simulink model "Test_measurement_script"  (R2019b)
settings: Solver=FixedStepAuto  StartTime=0.0  StopTime=10.0  RelTol=1e-3
PostLoadFcn:
  | if any(exist('dsrtsu_mdlpostloadfcn', 'file') ~= 0), dsrtsu_mdlpostloadfcn('Execute', bdroot); end
values from neighbouring files (symbols this model uses):
  UseUserDefinedBallReference = 1    [LQG_ball.m]    (also in LQG_plate_ball.m; LQR_ball.m; PerformExperiment_CompareModelWithMeasurement.m = 0; Template_PerformExperiment.m = 0)
  UseUserDefinedPlateReference = 1    [LQG_ball.m]    (also in LQG_plate_ball.m; LQR_ball.m; PerformExperiment_CompareModelWithMeasurement.m; Template_PerformExperiment.m = 0)
settings Model: DSRTSU_INTERNAL_RTI_VER=570  DSRTSU_INTERNAL_RTI_TYPE=rti1202  Creator=Duin home  LastModifiedBy=20201073
settings HardwareCC: ProdBitPerPointer=32  ProdBitPerSizeT=32  ProdBitPerPtrDiffT=32  ProdLargestAtomicInteger=Integer  ProdEndianess=BigEndian  ProdWordSize=32  ProdLongLongMode=on  ProdHWDeviceType=Custom Processor->Custom  TargetIntDivRoundTo=Zero  TargetEndianess=BigEndian  TargetHWDeviceType=Custom Processor->Custom
settings SFSimCC: MATLABDynamicMemAlloc=off
settings RTWCC: Description=dSPACE DS1202 Hardware Platform  SystemTargetFile=rti1202.tlc  MakeCommand=make_rti  TemplateMakefile=rti1202.tmf
settings STFCustomTargetCC: ParMdlRefBuildCompliant=on  SystemTargetFile=rti1202.tlc
settings GRTTargetCC: TargetLangStandard=C89/C90 (ANSI)  CompOptLevelCompliant=off  ConcurrentExecutionCompliant=off  CombineOutputUpdateFcns=off  MatFileLogging=off  CPPClassGenCompliant=off  UseToolchainInfoCompliant=off

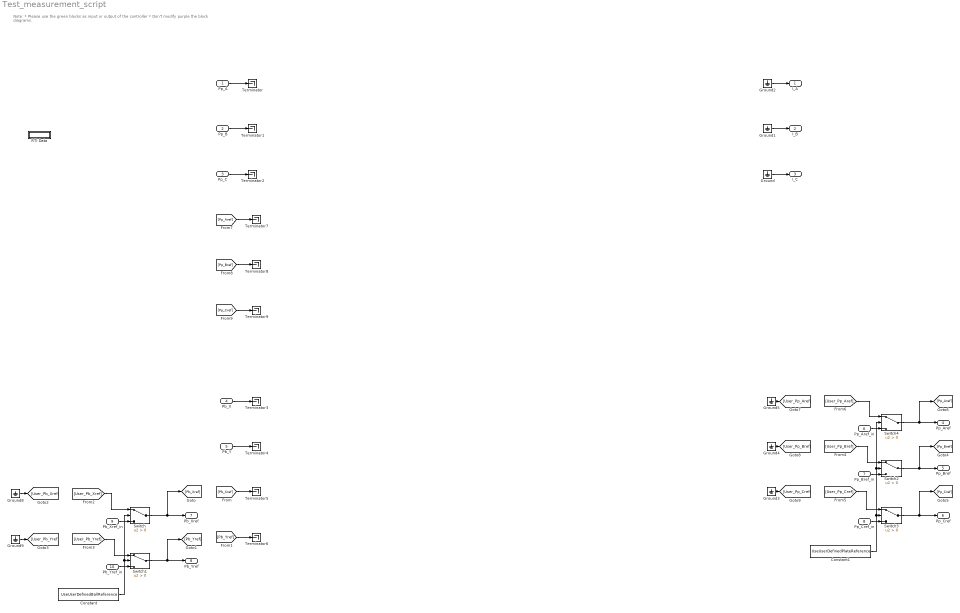
== system Test_measurement_script ==
  note: Note:
      | * Please use the green blocks as input or output of the controller
      | * Don't modify purple the block diagrams.
  Pp_A : Inport
  Pp_B : Inport  Port=2
  Pp_C : Inport  Port=3
  Pb_X : Inport  Port=4
  Pb_Y : Inport  Port=5
  Pp_Aref_in : Inport  Port=6
  Pp_Bref_in : Inport  Port=7
  Pp_Cref_in : Inport  Port=8
  Pb_Xref_in : Inport  Port=9
  Pb_Yref_in : Inport  Port=10
  Constant : Constant  Value=UseUserDefinedBallReference
  Constant1 : Constant  Value=UseUserDefinedPlateReference
  Ground{,1..5,8..9} (8 alike) : Ground
  RTI Data : Subsystem  Tag=struct('RTIDataServer',struct('RTIDataServerVs','2','RTIModelDescription','struct(''main'',''Test_measurement_script'',''sub'',''Test_measurement_script'',''isMp'',0)'))  LoadFcn="if exist('rtidc'), try,  rtidc('DataHostBlockClbLoad', gcbh); catch, disp(['Warning: ''LoadFcn'' for RTI Data block failed: ' lasterr]); end, end,"  mask(RTI_DATA_HOST){}
      mask help:
      | RTI Data Block.
      | This block is used by RTI to store internal model-dependent data.
      | Please keep this block on the root level of the model. Deleting this block will result in data loss.
      |
      | NEVER DELETE OR COPY THIS BLOCK!
      settings: CopyFcn="if exist('rtidc'), try,  rtidc('DataHostBlockClbCopy', gcbh); catch, disp(['Warning: ''CopyFcn'' for RTI Data block failed: ' lasterr]); end, end,"  DeleteFcn="if exist('rtidc'), try,  rtidc('DataHostBlockClbDelete', gcbh); catch, disp(['Warning: ''DeleteFcn'' for RTI Data block failed: ' lasterr]); end, end,"  ModelCloseFcn="if exist('rtidc'), try,  rtidc('DataHostBlockClbModelClose', gcbh); catch, disp(['Warning: ''ModelCloseFcn'' for RTI Data block failed: ' lasterr]); end, end,"  PreSaveFcn="if exist('rtidc'), try,  rtidc('DataHostBlockClbPreSave', gcbh); catch, disp(['Warning: ''PreSaveFcn'' for RTI Data block failed: ' lasterr]); end, end,"  PostSaveFcn="if exist('rtidc'), try,  rtidc('DataHostBlockClbPostSave', gcbh); catch, disp(['Warning: ''PostSaveFcn'' for RTI Data block failed: ' lasterr]); end, end,"  NameChangeFcn="if exist('rtidc'), try,  rtidc('DataHostBlockClbNameChange', gcbh); catch, disp(['Warning: ''NameChangeFcn'' for RTI Data block failed: ' lasterr]); end, end,"
      mask Help:
      | RTI Data Block.
      | This block is used by RTI to store internal model-dependent data.
      | Please keep this block on the root level of the model. Deleting this block will result in data loss.
      | 
      | NEVER DELETE OR COPY THIS BLOCK!
      mask Display:
      | text(0.5, 0.5, 'RTI Data', 'HorizontalAlignment', 'center');
      | plot([1 0]);
  Switch{,1..4} (5 alike) : Switch  Criteria=u2 > Threshold
  Terminator{,1..9} (10 alike) : Terminator
  I_A : Outport
  I_B : Outport  Port=2
  I_C : Outport  Port=3
  Pp_Aref : Outport  Port=4
  Pp_Bref : Outport  Port=5
  Pp_Cref : Outport  Port=6
  Pb_Xref : Outport  Port=7
  Pb_Yref : Outport  Port=8
  wires:
  Pp_A/1 -> Terminator/1
  Pp_B/1 -> Terminator1/1
  Pp_C/1 -> Terminator2/1
  Pb_X/1 -> Terminator3/1
  Pb_Y/1 -> Terminator4/1
  Ground/1 -> I_C/1
  Ground1/1 -> I_B/1
  Ground2/1 -> I_A/1
  Ground3/1 -> [User_Pp_Cref]
  Ground4/1 -> [User_Pp_Bref]
  Ground5/1 -> [User_Pp_Aref]
  Pb_Xref_in/1 -> Switch/3
  Pb_Yref_in/1 -> Switch1/3
  Switch1/1 -> [Pb_Yref], Pb_Yref/1
  Switch/1 -> [Pb_Xref], Pb_Xref/1
  [User_Pb_Xref] -> Switch/1
  [User_Pb_Yref] -> Switch1/1
  Constant/1 -> Switch/2, Switch1/2
  Ground8/1 -> [User_Pb_Xref]
  Ground9/1 -> [User_Pb_Yref]
  [Pb_Yref] -> Terminator6/1
  [Pb_Xref] -> Terminator5/1
  Pp_Bref_in/1 -> Switch2/3
  [User_Pp_Bref] -> Switch2/1
  Switch3/1 -> [Pp_Cref], Pp_Cref/1
  Switch2/1 -> [Pp_Bref], Pp_Bref/1
  Pp_Cref_in/1 -> Switch3/3
  Constant1/1 -> Switch4/2, Switch2/2, Switch3/2
  [User_Pp_Cref] -> Switch3/1
  [User_Pp_Aref] -> Switch4/1
  Pp_Aref_in/1 -> Switch4/3
  Switch4/1 -> [Pp_Aref], Pp_Aref/1
  [Pp_Bref] -> Terminator8/1
  [Pp_Aref] -> Terminator7/1
  [Pp_Cref] -> Terminator9/1

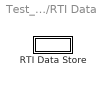
== system Test_measurement_script/RTI Data ==
  RTI Data Store : Subsystem  Tag=struct('private',struct('version',struct('dsVer',uint32(2),'dsVerCreation',uint32(2),'RTI',struct('ver','7.15','type','RTI1202')),'access',struct('type','Model','isPerm',1,'created',['01-Jun-2021 19:32:05'],'modified',['01-Jun-2021 19:37:03'],'location','')),'public',struct('main',struct('data',[]),'sub',struct('name','','data',[])))  mask(RTI_DATA_STORE){}
      mask help:
      | RTI Data Store Block. This block is used by RTI to store internal model dependent data. Deleting this block will result in data loss.
      |
      | NEVER DELETE, COPY, OR MODIFY THIS BLOCK!
      mask Help:
      | RTI Data Store Block. This block is used by RTI to store internal model dependent data. Deleting this block will result in data loss.
      | 
      | NEVER DELETE, COPY, OR MODIFY THIS BLOCK!
      mask Display: text(0.5, 0.5, ' ', 'HorizontalAlignment', 'center');

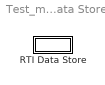
== system Test_measurement_script/RTI Data/RTI Data Store ==
  RTI Data Store : Subsystem  mask(RTI_DATA_STORE){}
      mask help:
      | RTI Data Store Block. This block is used by RTI to store internal model dependent data. Deleting this block will result in data loss.
      |
      | NEVER DELETE, COPY, OR MODIFY THIS BLOCK!
      mask Help:
      | RTI Data Store Block. This block is used by RTI to store internal model dependent data. Deleting this block will result in data loss.
      | 
      | NEVER DELETE, COPY, OR MODIFY THIS BLOCK!
      mask Display: text(0.5, 0.5, ' ', 'HorizontalAlignment', 'center');

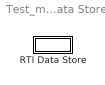
== system Test_measurement_script/RTI Data/RTI Data Store/RTI Data Store ==
  RTI Data Store : Subsystem  mask(RTI_DATA_STORE){}
      mask help:
      | RTI Data Store Block. This block is used by RTI to store internal model dependent data. Deleting this block will result in data loss.
      |
      | NEVER DELETE, COPY, OR MODIFY THIS BLOCK!
      mask Help:
      | RTI Data Store Block. This block is used by RTI to store internal model dependent data. Deleting this block will result in data loss.
      | 
      | NEVER DELETE, COPY, OR MODIFY THIS BLOCK!
      mask Display: text(0.5, 0.5, ' ', 'HorizontalAlignment', 'center');

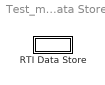
== system Test_measurement_script/RTI Data/RTI Data Store/RTI Data Store/RTI Data Store ==
  RTI Data Store : Subsystem  mask(RTI_DATA_STORE){}
      mask help:
      | RTI Data Store Block. This block is used by RTI to store internal model dependent data. Deleting this block will result in data loss.
      |
      | NEVER DELETE, COPY, OR MODIFY THIS BLOCK!
      mask Help:
      | RTI Data Store Block. This block is used by RTI to store internal model dependent data. Deleting this block will result in data loss.
      | 
      | NEVER DELETE, COPY, OR MODIFY THIS BLOCK!
      mask Display: text(0.5, 0.5, ' ', 'HorizontalAlignment', 'center');

== system Test_measurement_script/RTI Data/RTI Data Store/RTI Data Store/RTI Data Store/RTI Data Store ==
